simulink model "Dynamic_model"  (R2018a)
settings: Solver=VariableStepAuto  StartTime=0.0  StopTime=10.0  RelTol=1e-3
values from neighbouring files (symbols this model uses):
  Fv_longi = 0.0    [Dynamic_model.sldd]
  Fv_rot = 0.0    [Dynamic_model.sldd]
  L_robot = 0.25    [Dynamic_model.sldd]
  l_wheel = 0.225    [Dynamic_model.sldd]
  M_robot = 7.0    [Dynamic_model.sldd]
libraries: simulink x2
settings Model: DataDictionary=Dynamic_model.sldd  Creator=hugo  LastModifiedBy=hugo

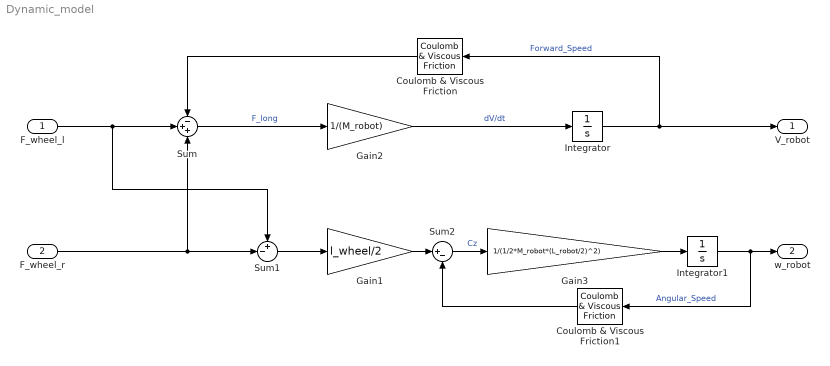
== system Dynamic_model ==
  F_wheel_l : Inport
  F_wheel_r : Inport  Port=2
  Coulomb & Viscous Friction : simulink/Discontinuities/Coulomb & Viscous Friction  offset=Fs_longi  gain=Fv_longi
      settings: SourceProductName=Simulink
  Coulomb & Viscous Friction1 : simulink/Discontinuities/Coulomb & Viscous Friction  offset=Fs_rot  gain=Fv_rot
      settings: SourceProductName=Simulink
  Gain1 : Gain  Gain=l_wheel/2
  Gain2 : Gain  Gain=1/(M_robot)
  Gain3 : Gain  Gain=1/(1/2*M_robot*(L_robot/2)^2)
  Integrator : Integrator  ContinuousStateAttributes='Forward_Speed'
  Integrator1 : Integrator  ContinuousStateAttributes='Vitesse_Longitudinale'
  Sum : Sum  Inputs=-++
  Sum1 : Sum  Inputs=+-|
  Sum2 : Sum  Inputs=|+-
  V_robot : Outport
  w_robot : Outport  Port=2
  wires:
  F_wheel_r/1 -> Sum1/2, Sum/3
  Sum2/1 -> Gain3/1  "Cz"
  Coulomb & Viscous Friction/1 -> Sum/1
  Gain3/1 -> Integrator1/1
  Coulomb & Viscous Friction1/1 -> Sum2/2
  Gain1/1 -> Sum2/1
  F_wheel_l/1 -> Sum1/1, Sum/2
  Integrator1/1 -> Coulomb & Viscous Friction1/1, w_robot/1  "Angular_Speed"
  Gain2/1 -> Integrator/1  "dV/dt"
  Sum/1 -> Gain2/1  "F_long"
  Integrator/1 -> Coulomb & Viscous Friction/1, V_robot/1  "Forward_Speed"
  Sum1/1 -> Gain1/1
